simulink model "FB_Controller_UCS"  (R2025b)
settings: Solver=FixedStepDiscrete  StartTime=0.0  StopTime=tspan  FixedStep=dt_sim  RelTol=rel_tol  AbsTol=abs_tol
undefined symbols (not defined in the file): camHardwareDistK, Cimub, const_voltage, dt_control, dt_data, dt_dvl_drr, dt_dvl_vr, dt_sample, dvl, gate1_Pose, initial_joystick_mode_enabled_flag, M_WorldToUCS, manateeOriginPose, pathPoses, redSlalomPoses, rel_CamPose_B, rel_CamPose_B_UCS, rel_CamPose_L, rel_CamPose_L_UCS, rel_CamPose_R, rel_CamPose_R_UCS, save_camera_feed_flag, searchRescueEmojiPose, Sim3dSensor, surveyRepairEmojiPose, use_true_state_flag, whiteSlalomPoses
libraries: sim3dlib x30, visionsinks x3, sim3dcameralib x3, mspsensorlib x1
settings Model: Creator=koryh  LastModifiedBy=Liam

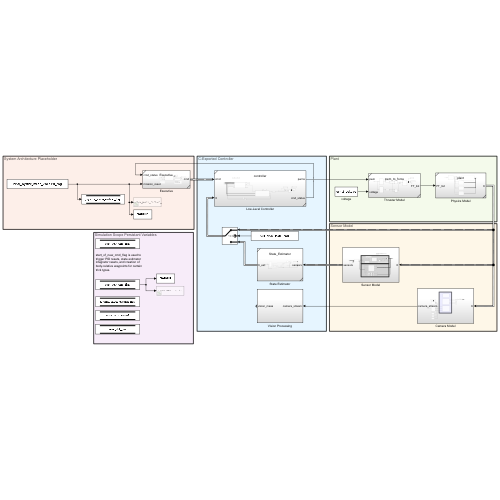
[thumbnail: Simulink's stored preview of the top-level diagram]
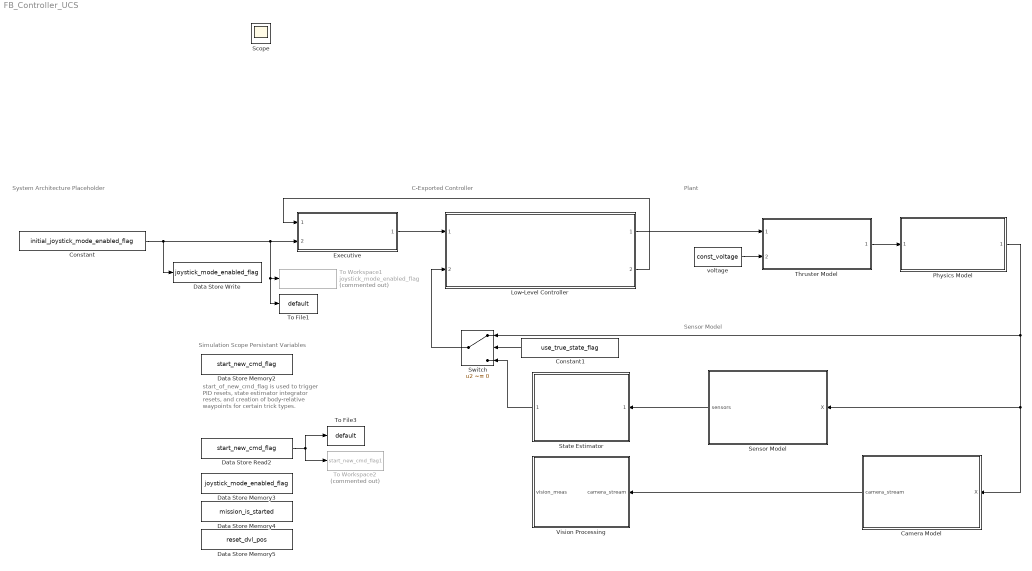
== system FB_Controller_UCS ==
  note: System Architecture Placeholder
  note: Sensor Model
  note: Plant
  note: C-Exported Controller
  note: Simulation Scope Persistant Variables
  note: start_of_new_cmd_flag is used to trigger PID resets, state estimator integrator resets, and creation of body-relative waypoints for certain trick types.
  Camera Model : Subsystem
  Constant : Constant  Value=initial_joystick_mode_enabled_flag
  Constant1 : Constant  Value=use_true_state_flag
  Data Store Memory2 : DataStoreMemory  DataStoreName=start_new_cmd_flag  WriteAfterWriteMsg=warning  InitialValue=true  ShowAdditionalParam=off  OutDataTypeStr=boolean
  Data Store Memory3 : DataStoreMemory  DataStoreName=joystick_mode_enabled_flag  WriteAfterWriteMsg=warning  InitialValue=initial_joystick_mode_enabled_flag  ShowAdditionalParam=off  OutDataTypeStr=boolean
  Data Store Memory4 : DataStoreMemory  DataStoreName=mission_is_started  WriteAfterWriteMsg=warning  InitialValue=false  ShowAdditionalParam=off  OutDataTypeStr=boolean
  Data Store Memory5 : DataStoreMemory  DataStoreName=reset_dvl_pos  WriteAfterWriteMsg=warning  InitialValue=false  ShowAdditionalParam=off  OutDataTypeStr=boolean
  Data Store Read2 : DataStoreRead  DataStoreName=start_new_cmd_flag  IndexOptions=Index vector (dialog)  Indices=1  OutputSizes=1
  Data Store Write : DataStoreWrite  DataStoreName=joystick_mode_enabled_flag  IndexOptions=Index vector (dialog)  Indices=1  OutputSizes=1
  Executive : Subsystem  ReferencedSubsystem=Executive
  Low-Level Controller : Subsystem  ReferencedSubsystem=controller
  Physics Model : Subsystem  ReferencedSubsystem=plant
  Sensor Model : Subsystem
  State Estimator : Subsystem  ReferencedSubsystem=State_Estimator
  Switch : Switch  Criteria=u2 ~= 0  SaturateOnIntegerOverflow=off  InputSameDT=off
  Thruster Model : Subsystem  ReferencedSubsystem=pwm_to_force
  To File1 : ToFile  Filename=default  MatrixName=joystick_mode_enabled_flag  SaveFormat=Timeseries  SampleTime=dt_data
  To File3 : ToFile  Filename=default  MatrixName=start_new_cmd_flag  SaveFormat=Timeseries
  To Workspace1 : ToWorkspace  Commented=on  VariableName=joystick_mode_enabled_flag  SaveFormat=Timeseries  SampleTime=dt_data
  To Workspace2 : ToWorkspace  Commented=on  VariableName=start_new_cmd_flag1  SaveFormat=Timeseries  SampleTime=dt_data
  Vision Processing : Subsystem
  voltage : Constant  Value=const_voltage
  Scope : Scope
      settings: ActiveDisplayYMinimum=-0.048832566475369238  ActiveDisplayYMaximum=0.79721663606048965
  wires:
  voltage/1 -> Thruster Model/2
  Low-Level Controller/1 -> Thruster Model/1
  Thruster Model/1 -> Physics Model/1
  Executive/1 -> Low-Level Controller/1
  Low-Level Controller/2 -> Executive/1
  Physics Model/1 -> Sensor Model/1(X), Camera Model/1(X), Switch/1
  Camera Model/1(camera_stream) -> Vision Processing/1(camera_stream)
  Sensor Model/1(sensors) -> State Estimator/1
  Switch/1 -> Low-Level Controller/2
  Constant1/1 -> Switch/2
  State Estimator/1 -> Switch/3
  Constant/1 -> Data Store Write/1, To File1/1, To Workspace1/1, Executive/2
  Data Store Read2/1 -> To File3/1, To Workspace2/1

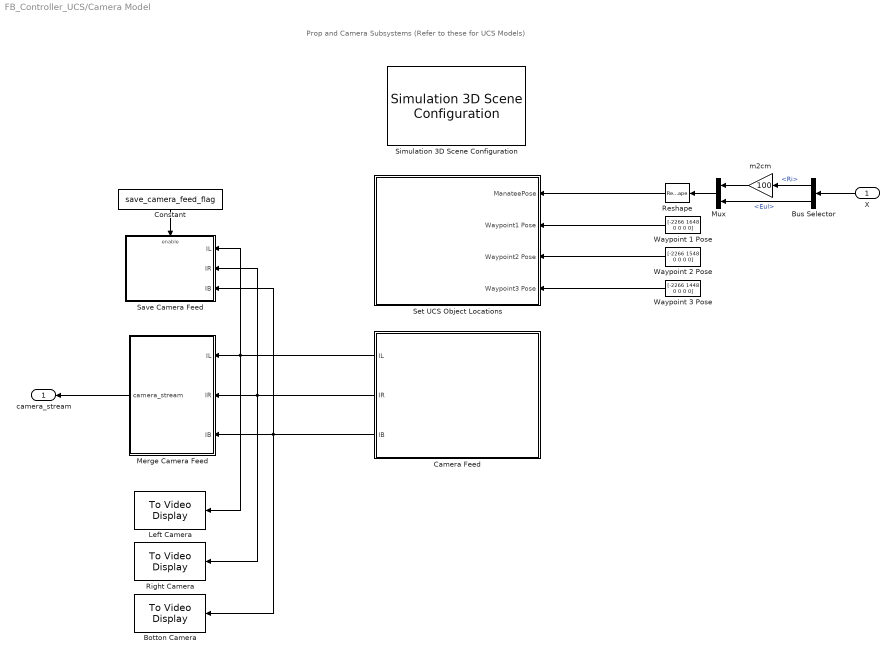
== system FB_Controller_UCS/Camera Model ==
  note: Prop and Camera Subsystems (Refer to these for UCS Models)
  X : Inport
  Botton Camera : visionsinks/To Video Display  windowSizeMode=Normal  openAtMdlStart=off  fullScreen=off  videoWindowX=536805376  videoWindowY=536805376  saveWindowSize=off  videoWindowWidth=1491  videoWindowHeight=834  inputColorFormat=RGB  inputType=Obsolete  imagePorts=One multidimensional signal  OutputDevice=On-screen video monitor  dataOrg=Column-major  isWindowOpen=off
  Bus Selector : BusSelector  OutputSignals=Ri,Eul
  Camera Feed : Subsystem  Priority=1
  Constant : Constant  Value=save_camera_feed_flag
  Left Camera : visionsinks/To Video Display  windowSizeMode=Normal  openAtMdlStart=off  fullScreen=off  videoWindowX=536805376  videoWindowY=536805376  saveWindowSize=off  videoWindowWidth=1491  videoWindowHeight=834  inputColorFormat=RGB  inputType=Obsolete  imagePorts=One multidimensional signal  OutputDevice=On-screen video monitor  dataOrg=Column-major  isWindowOpen=off
  Merge Camera Feed : MATLAB Function  TreatAsAtomicUnit=on
  Mux : Mux  Inputs=2
  Reshape : Reshape  OutputDimensionality=Row vector (2-D)
  Right Camera : visionsinks/To Video Display  windowSizeMode=Normal  openAtMdlStart=off  fullScreen=off  videoWindowX=536805376  videoWindowY=536805376  saveWindowSize=off  videoWindowWidth=1491  videoWindowHeight=834  inputColorFormat=RGB  inputType=Obsolete  imagePorts=One multidimensional signal  OutputDevice=On-screen video monitor  dataOrg=Column-major  isWindowOpen=off
  Save Camera Feed : Subsystem  TreatAsAtomicUnit=on
  Set UCS Object Locations : Subsystem  Priority=1
  Simulation 3D Scene Configuration : sim3dlib/Simulation 3D Scene Configuration  Priority=0  ProjectFormat=Unreal Executable  SceneDesc=Straight road  ProjectName=C:\Users\Liam\OneDrive\Documents\GitHub\SimulinkPlant\DROP UCS PACKAGED BUILD HERE\EllingtonPoolSim.exe  ScenePath=/Game/Olympic_Pool_Course  UEProjPath=C:\Users\Liam\OneDrive\Documents\GitHub\Vision_Sim\Unreal\UnrealProjects\SimulinkCoSimulation\EllingtonPoolSim\EllingtonPoolSim.uproject  EnableOpenDRIVE=off  vehTagList={'Custom';'Scene Origin'}  vehTag=Scene Origin  AttachedCameraRelativeTranslation=[0 0 0]  FreeCameraDefaultInitialTranslation=[-6, 0, 2]  AttachedCameraRelativeRotation=[0 0 0]  FreeCameraDefaultInitialRotation=[0, -15, 0]  ViewpointName=Custom  FreeCameraInitialTranslation=[0, 0, 0]  ViewpointTranslation=[0 0 0]  FreeCameraInitialRotation=[0, 0, 0]  ViewpointRotation=[0 0 0]  OpVisEn=off  Ts=dt_sample  EnableWindow=off  EnableRemoteAccess=off  EnableWeather=off  SunAzimuth=90  SunAltitude=40.0  EnableGeospatialSun=off  Latitude=0  Longitude=0  Date=2023-01-01  Time=10:30:00  GeoTimeZone=-5.0  SunDaylightSaving=off  wind=1  clouds=10  EnableVolumetricClouds=off  CloudCoverage=0  CloudAltitude=6  fog=0  rain=0  RaindropsEffect=off  SnowDensity=0  EnableGeospatial=off  TilesetSource=Earth terrain  UseTrueOrigin=off  OriginHeight=200  OriginLatitude=40.744652  OriginLongitude=-73.988864  MapStyle=Aerial  AdditionalAssetIDs=[]  UseAdvancedSunSky=off  SolarTime=11  TimeZone=-5  Day=21  Month=9  Year=2022  UseDaylightSavingTime=on  DSTStartDay=10  DSTStartMonth=3  DSTEndDay=3  DSTEndMonth=11  DSTSwitchHour=2  sensorTag=MainCamera1  sensorId=1  sensorName=MainCamera1  mountLoc=Origin  offsetFlag=off  tmountOffset=[0, 0, 0]  rmountOffset=[0, 0, 0]  HorizontalResolution=1280  VerticalResolution=720  HorizontalFOV=60  mountPoint=[0 0 0]  mountOrientation=[0 0 0]  aMode=3  ID=1  GeoTrigger=Inactive  ViewNameList={'Custom'}  ViewTranslationList={'[0 0 0]'}  ViewRotationList={'[0 0 0]'}
      settings: LibrarySourceBlock=drivingsim3d/Simulation 3D Scene Configuration
  Waypoint 1 Pose : Constant  Value=[-2266 1648 0 0 0 0]
  Waypoint 2 Pose : Constant  Value=[-2266 1548 0 0 0 0]
  Waypoint 3 Pose : Constant  Value=[-2266 1448 0 0 0 0]
  m2cm : Gain  Gain=100
  camera_stream : Outport
  wires:
  X/1 -> Bus Selector/1
  Bus Selector/1 -> m2cm/1  "<Ri>"
  Bus Selector/2 -> Mux/2  "<Eul>"
  Mux/1 -> Reshape/1
  m2cm/1 -> Mux/1
  Reshape/1 -> Set UCS Object Locations/1(ManateePose)
  Waypoint 1 Pose/1 -> Set UCS Object Locations/2(Waypoint1 Pose)
  Waypoint 2 Pose/1 -> Set UCS Object Locations/3(Waypoint2 Pose)
  Waypoint 3 Pose/1 -> Set UCS Object Locations/4(Waypoint3 Pose)
  Camera Feed/1(IL) -> Save Camera Feed/1(IL), Merge Camera Feed/1(IL), Left Camera/1
  Camera Feed/2(IR) -> Save Camera Feed/2(IR), Merge Camera Feed/2(IR), Right Camera/1
  Camera Feed/3(IB) -> Save Camera Feed/3(IB), Merge Camera Feed/3(IB), Botton Camera/1
  Merge Camera Feed/1(camera_stream) -> camera_stream/1
  Constant/1 -> Save Camera Feed/Enable

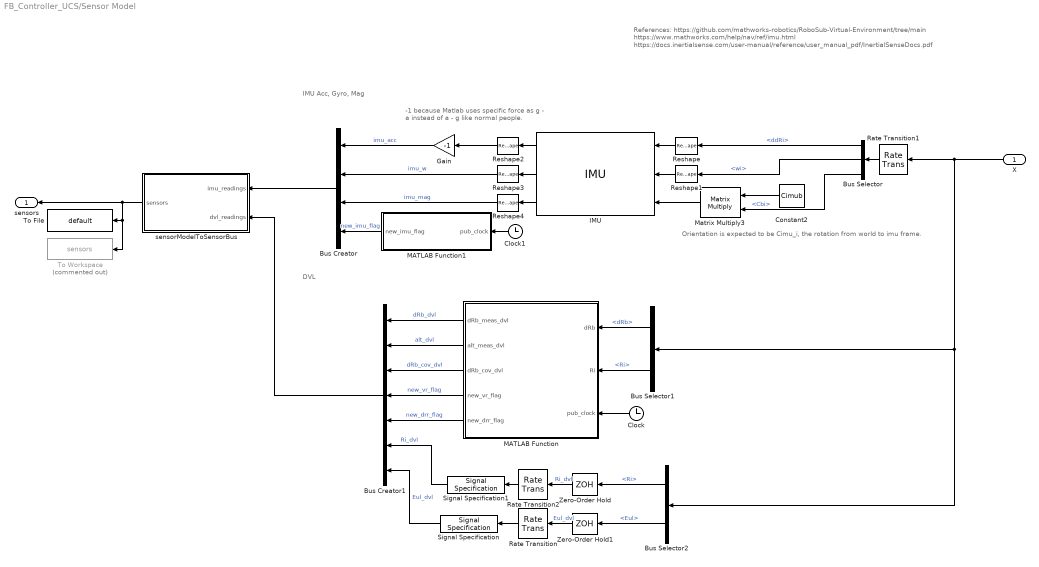
== system FB_Controller_UCS/Sensor Model ==
  note: IMU Acc, Gyro, Mag
  note: -1 because Matlab uses specific force as
      |  g - a instead of a - g like normal people.
  note: Orientation is expected to be Cimu_i, the rotation from world to imu frame.
  note: References:
      | https://github.com/mathworks-robotics/RoboSub-Virtual-Environment/tree/main
      | https://www.mathworks.com/help/nav/ref/imu.html
      | https://docs.inertialsense.com/user-manual/reference/user_manual_pdf/InertialSenseDocs.pdf
  note: DVL
  X : Inport  OutDataTypeStr=Bus: X_bus  SampleTime=dt_control
  Bus Creator : BusCreator  Inputs=4  OutDataTypeStr=Bus: imu_bus
  Bus Creator1 : BusCreator  Inputs=7  OutDataTypeStr=Bus: dvl_bus
  Bus Selector : BusSelector  OutputSignals=ddRi,wi,Cbi
  Bus Selector1 : BusSelector  OutputSignals=dRb,Ri
  Bus Selector2 : BusSelector  OutputSignals=Ri,Eul
  Clock : Clock
  Clock1 : Clock
  Constant2 : Constant  Value=Cimub
  Gain : Gain  Gain=-1
  IMU : mspsensorlib/IMU  DispRefFrame=NED  TemperaturePort=off  Temperature=imu.T  MagneticFieldPort=off  MagneticFieldNED=imu.Bi  MagneticFieldENU=[ -2.4169, 27.5550, 16.0849 ]  SeedDouble=67  SimulateUsing=Interpreted execution  AccelParamsMeasurementRange=imu.acc.meas_range  AccelParamsResolution=imu.acc.res  AccelParamsConstantBias=imu.acc.const_bias  AccelParamsAxesMisalignment=imu.acc.axes_skew  AccelParamsNoiseDensity=imu.acc.vel_rand_walk  AccelParamsBiasInstability=imu.acc.bias_inst  AccelParamsBiasInstabilityNumerator=imu.acc.bias_inst_num_coeffs  AccelParamsBiasInstabilityDenominator=imu.acc.bias_inst_den_coeffs  AccelParamsRandomWalk=imu.acc.acc_rand_walk  AccelParamsNoiseType=double-sided  AccelParamsTemperatureBias=imu.acc.temp_bias  AccelParamsTemperatureScaleFactor=imu.acc.temp_scale_factor  GyroParamsMeasurementRange=imu.gyro.max_read  GyroParamsResolution=imu.gyro.res  GyroParamsConstantBias=imu.gyro.const_bias  GyroParamsAxesMisalignment=imu.gyro.axes_skew  GyroParamsAccelerationBias=imu.gyro.bias_from_acc  GyroParamsNoiseDensity=imu.gyro.angle_rand_walk  GyroParamsBiasInstability=imu.gyro.bias_inst  GyroParamsBiasInstabilityNumerator=imu.gyro.bias_inst_filter_num_coeffs  GyroParamsBiasInstabilityDenominator=imu.gyro.bias_inst_filter_den_coeffs  GyroParamsRandomWalk=imu.gyro.rate_rand_walk  GyroParamsNoiseType=double-sided  GyroParamsTemperatureBias=imu.gyro.temp_bias  GyroParamsTemperatureScaleFactor=imu.gyro.temp_scale_factor  MagParamsMeasurementRange=imu.mag.max_read  MagParamsResolution=imu.mag.res  MagParamsConstantBias=imu.mag.const_bias  MagParamsAxesMisalignment=imu.mag.axes_skew  MagParamsNoiseDensity=imu.mag.white_noise_psd  MagParamsBiasInstability=imu.mag.bias_inst  MagParamsBiasInstabilityNumerator=imu.mag.bias_inst_filter_num_coeffs  MagParamsBiasInstabilityDenominator=imu.mag.bias_isnt_filter_den_coeffs  MagParamsRandomWalk=imu.mag.rand_walk  MagParamsNoiseType=double-sided  MagParamsTemperatureBias=imu.mag.temp_bias  MagParamsTemperatureScaleFactor=imu.mag.temp_scale_factor
  MATLAB Function : MATLAB Function  TreatAsAtomicUnit=on
  MATLAB Function1 : MATLAB Function  TreatAsAtomicUnit=on
  Matrix Multiply3 : Product  Multiplication=Matrix(*)
  Rate Transition : RateTransition  Deterministic=off  OutPortSampleTime=dt_control
  Rate Transition1 : RateTransition  OutPortSampleTime=dt_imu
  Rate Transition2 : RateTransition  Deterministic=off  OutPortSampleTime=dt_control
  Reshape : Reshape  OutputDimensionality=Row vector (2-D)
  Reshape1 : Reshape  OutputDimensionality=Row vector (2-D)
  Reshape2 : Reshape  OutputDimensionality=Column vector (2-D)
  Reshape3 : Reshape  OutputDimensionality=Column vector (2-D)
  Reshape4 : Reshape  OutputDimensionality=Column vector (2-D)
  Signal Specification : SignalSpecification  SampleTime=dt_control
  Signal Specification1 : SignalSpecification  SampleTime=dt_control
  To File : ToFile  Filename=default  MatrixName=sensors  SaveFormat=Timeseries  SampleTime=dt_data
  To Workspace : ToWorkspace  Commented=on  VariableName=sensors  SaveFormat=Timeseries  SampleTime=dt_data
  Zero-Order Hold : ZeroOrderHold  SampleTime=dt_dvl_drr
  Zero-Order Hold1 : ZeroOrderHold  SampleTime=dt_dvl_drr
  sensorModelToSensorBus : MATLAB Function  TreatAsAtomicUnit=on
  sensors : Outport  OutDataTypeStr=Bus: sensor_bus  SampleTime=dt_control
  wires:
  X/1 -> Rate Transition1/1, Bus Selector2/1, Bus Selector1/1
  Reshape/1 -> IMU/1
  Bus Selector/2 -> Reshape1/1  "<wi>"
  IMU/1 -> Reshape2/1
  IMU/2 -> Reshape3/1
  IMU/3 -> Reshape4/1
  Reshape1/1 -> IMU/2
  Bus Selector/1 -> Reshape/1  "<ddRi>"
  Matrix Multiply3/1 -> IMU/3
  Constant2/1 -> Matrix Multiply3/1
  Bus Selector/3 -> Matrix Multiply3/2  "<Cbi>"
  Reshape2/1 -> Gain/1
  Bus Selector1/1 -> MATLAB Function/1(dRb)  "<dRb>"
  Bus Selector1/2 -> MATLAB Function/2(Ri)  "<Ri>"
  sensorModelToSensorBus/1(sensors) -> sensors/1, To Workspace/1, To File/1
  Bus Selector2/2 -> Zero-Order Hold1/1  "<Eul>"
  Rate Transition1/1 -> Bus Selector/1
  Clock/1 -> MATLAB Function/3(pub_clock)
  Clock1/1 -> MATLAB Function1/1(pub_clock)
  Gain/1 -> Bus Creator/1  "imu_acc"
  Reshape3/1 -> Bus Creator/2  "imu_w"
  Reshape4/1 -> Bus Creator/3  "imu_mag"
  MATLAB Function1/1(new_imu_flag) -> Bus Creator/4  "new_imu_flag"
  MATLAB Function/1(dRb_meas_dvl) -> Bus Creator1/1  "dRb_dvl"
  MATLAB Function/2(alt_meas_dvl) -> Bus Creator1/2  "alt_dvl"
  MATLAB Function/3(dRb_cov_dvl) -> Bus Creator1/3  "dRb_cov_dvl"
  MATLAB Function/4(new_vr_flag) -> Bus Creator1/4  "new_vr_flag"
  MATLAB Function/5(new_drr_flag) -> Bus Creator1/5  "new_drr_flag"
  Bus Creator/1 -> sensorModelToSensorBus/1(imu_readings)
  Bus Creator1/1 -> sensorModelToSensorBus/2(dvl_readings)
  Zero-Order Hold/1 -> Rate Transition2/1  "Ri_dvl"
  Signal Specification1/1 -> Bus Creator1/6  "Ri_dvl"
  Signal Specification/1 -> Bus Creator1/7  "Eul_dvl"
  Rate Transition/1 -> Signal Specification/1
  Rate Transition2/1 -> Signal Specification1/1
  Zero-Order Hold1/1 -> Rate Transition/1  "Eul_dvl"
  Bus Selector2/1 -> Zero-Order Hold/1  "<Ri>"

== system FB_Controller_UCS/Vision Processing ==
  camera_stream : Inport
  vision_meas : Outport

== system FB_Controller_UCS/Camera Model/Camera Feed ==
  Simulation 3D Manatee Bottom Camera : sim3dcameralib/Simulation 3D Camera  Priority=1  sensorTag=Sim3dSensor�  sensorId=1  sensorName=Sim3dSensor�  vehTagList={'Scene Origin'}  vehTag=Scene Origin  CoordinateSystem=Default  mountLoc=Origin  offsetFlag=on  tmountOffset=rel_CamPose_B_UCS(1:3) / 100  extTmount=off  rmountOffset=rel_CamPose_B(4:6)  extRmount=off  FocalLength=[2.97 / 0.0028, 2.97 / 0.0028]  OpticalCenter=[960, 540]  ImageSize=[1080, 1920]  RadialDistortion=[camHardwareDistK(1) camHardwareDistK(2) camHardwareDistK(5)]  TangentialDistortion=[camHardwareDistK(3) camHardwareDistK(4)]  SensorSkew=0  VisualizeFieldOfView=on  FieldOfViewRange=61  DepthOutportEnabled=off  SemanticOutportEnabled=off  TransformOutportEnabled=off  SampleTime=dt_sample  mountPoint=[0.23 0 -0.08]  mountOrientation=[0 -1.5707963267949 0]  aMode=5  ID=1
      settings: LibrarySourceBlock=sl3dlib/Simulation 3D/Sensors/Simulation 3D Camera
  Simulation 3D Manatee Left Camera : sim3dcameralib/Simulation 3D Camera  Priority=1  sensorTag=Sim3dSensor�  sensorId=2  sensorName=Sim3dSensor�  vehTagList={'Scene Origin'}  vehTag=Scene Origin  CoordinateSystem=Default  mountLoc=Origin  offsetFlag=on  tmountOffset=rel_CamPose_L_UCS(1:3) / 100  extTmount=off  rmountOffset=rel_CamPose_L(4:6)  extRmount=off  FocalLength=[2.97 / 0.0028, 2.97 / 0.0028]  OpticalCenter=[960, 540]  ImageSize=[1080, 1920]  RadialDistortion=[camHardwareDistK(1) camHardwareDistK(2) camHardwareDistK(5)]  TangentialDistortion=[camHardwareDistK(3) camHardwareDistK(4)]  SensorSkew=0  VisualizeFieldOfView=on  FieldOfViewRange=61  DepthOutportEnabled=off  SemanticOutportEnabled=off  TransformOutportEnabled=off  SampleTime=dt_sample  mountPoint=[0.38 -0.024 0.14]  mountOrientation=[0 0 0]  aMode=5  ID=2
      settings: LibrarySourceBlock=sl3dlib/Simulation 3D/Sensors/Simulation 3D Camera
  Simulation 3D Manatee Right Camera : sim3dcameralib/Simulation 3D Camera  Priority=1  sensorTag=Sim3dSensor�  sensorId=3  sensorName=Sim3dSensor�  vehTagList={'Scene Origin'}  vehTag=Scene Origin  CoordinateSystem=Default  mountLoc=Origin  offsetFlag=on  tmountOffset=rel_CamPose_R_UCS(1:3) / 100  extTmount=off  rmountOffset=rel_CamPose_R(4:6)  extRmount=off  FocalLength=[2.97 / 0.0028, 2.97 / 0.0028]  OpticalCenter=[960, 540]  ImageSize=[1080, 1920]  RadialDistortion=[camHardwareDistK(1) camHardwareDistK(2) camHardwareDistK(5)]  TangentialDistortion=[camHardwareDistK(3) camHardwareDistK(4)]  SensorSkew=0  VisualizeFieldOfView=on  FieldOfViewRange=61  DepthOutportEnabled=off  SemanticOutportEnabled=off  TransformOutportEnabled=off  SampleTime=dt_sample  mountPoint=[0.38 0.024 0.14]  mountOrientation=[0 0 0]  aMode=5  ID=3
      settings: LibrarySourceBlock=sl3dlib/Simulation 3D/Sensors/Simulation 3D Camera
  IL : Outport
  IR : Outport  Port=2
  IB : Outport  Port=3
  wires:
  Simulation 3D Manatee Left Camera/1 -> IL/1
  Simulation 3D Manatee Right Camera/1 -> IR/1
  Simulation 3D Manatee Bottom Camera/1 -> IB/1

== system FB_Controller_UCS/Camera Model/Save Camera Feed ==
  IL : Inport
  IR : Inport  Port=2
  IB : Inport  Port=3
  Enable : EnablePort
  To Workspace Bottom : ToWorkspace  Commented=on  VariableName=cameraBottom_Feed  SampleTime=dt_sample
  To Workspace Left : ToWorkspace  Commented=on  VariableName=cameraLeft_Feed  SampleTime=dt_sample
  To Workspace Right : ToWorkspace  Commented=on  VariableName=cameraRight_Feed  SampleTime=dt_sample
  wires:
  IL/1 -> To Workspace Left/1
  IR/1 -> To Workspace Right/1
  IB/1 -> To Workspace Bottom/1

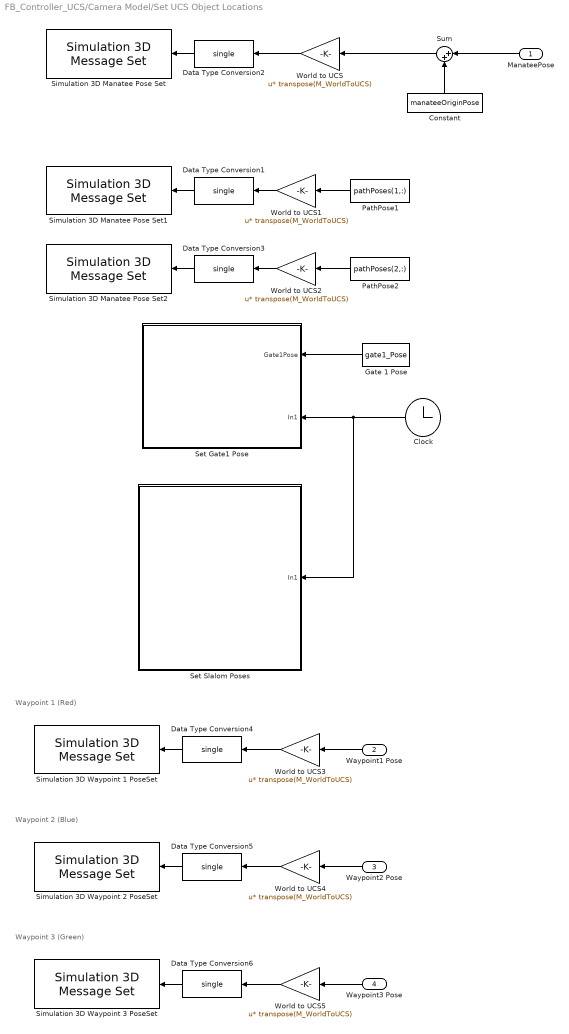
== system FB_Controller_UCS/Camera Model/Set UCS Object Locations ==
  note: Waypoint 1 (Red)
  note: Waypoint 2 (Blue)
  note: Waypoint 3 (Green)
  ManateePose : Inport
  Waypoint1 Pose : Inport  Port=2
  Waypoint2 Pose : Inport  Port=3
  Waypoint3 Pose : Inport  Port=4
  Clock : Clock
      settings: Decimation=dt_sample/dt_sim
  Constant : Constant  Value=manateeOriginPose
  Data Type Conversion{1..6} (6 alike) : DataTypeConversion  OutDataTypeStr=single  SaturateOnIntegerOverflow=off  RndMeth=Floor
  Gate 1 Pose : Constant  Value=gate1_Pose
  PathPose1 : Constant  Value=pathPoses(1,:)
  PathPose2 : Constant  Value=pathPoses(2,:)
  Set Gate1 Pose : Subsystem
  Set Slalom Poses : Subsystem
  Simulation 3D Manatee Pose Set : sim3dlib/Simulation 3D Message Set  Priority=-1  SigName=ManateePoseSet  Ts=dt_sample  aMode=0
      settings: LibrarySourceBlock=aerolibsim3d/Simulation 3D Message Set
  Simulation 3D Manatee Pose Set1 : sim3dlib/Simulation 3D Message Set  Priority=-1  SigName=Path1PoseSet  Ts=dt_sample  aMode=0
      settings: LibrarySourceBlock=aerolibsim3d/Simulation 3D Message Set
  Simulation 3D Manatee Pose Set2 : sim3dlib/Simulation 3D Message Set  Priority=-1  SigName=Path2PoseSet  Ts=dt_sample  aMode=0
      settings: LibrarySourceBlock=aerolibsim3d/Simulation 3D Message Set
  Simulation 3D Waypoint 1 PoseSet : sim3dlib/Simulation 3D Message Set  Priority=-1  SigName=Waypoint1PoseSet  Ts=dt_sample  aMode=0
      settings: LibrarySourceBlock=aerolibsim3d/Simulation 3D Message Set
  Simulation 3D Waypoint 2 PoseSet : sim3dlib/Simulation 3D Message Set  Priority=-1  SigName=Waypoint2PoseSet  Ts=dt_sample  aMode=0
      settings: LibrarySourceBlock=aerolibsim3d/Simulation 3D Message Set
  Simulation 3D Waypoint 3 PoseSet : sim3dlib/Simulation 3D Message Set  Priority=-1  SigName=Waypoint3PoseSet  Ts=dt_sample  aMode=0
      settings: LibrarySourceBlock=aerolibsim3d/Simulation 3D Message Set
  Sum : Sum  Inputs=|++
  World to UCS{,1..5} (6 alike) : Gain  Gain=transpose(M_WorldToUCS)  Multiplication=Matrix(u*K)
  wires:
  Gate 1 Pose/1 -> Set Gate1 Pose/1(Gate1Pose)
  Data Type Conversion2/1 -> Simulation 3D Manatee Pose Set/1
  World to UCS1/1 -> Data Type Conversion1/1
  Data Type Conversion1/1 -> Simulation 3D Manatee Pose Set1/1
  PathPose1/1 -> World to UCS1/1
  World to UCS2/1 -> Data Type Conversion3/1
  Data Type Conversion3/1 -> Simulation 3D Manatee Pose Set2/1
  PathPose2/1 -> World to UCS2/1
  Clock/1 -> Set Slalom Poses/1(In1), Set Gate1 Pose/2(In1)
  World to UCS/1 -> Data Type Conversion2/1
  Waypoint1 Pose/1 -> World to UCS3/1
  Data Type Conversion4/1 -> Simulation 3D Waypoint 1 PoseSet/1
  World to UCS3/1 -> Data Type Conversion4/1
  Waypoint2 Pose/1 -> World to UCS4/1
  Data Type Conversion5/1 -> Simulation 3D Waypoint 2 PoseSet/1
  World to UCS4/1 -> Data Type Conversion5/1
  World to UCS5/1 -> Data Type Conversion6/1
  Waypoint3 Pose/1 -> World to UCS5/1
  Data Type Conversion6/1 -> Simulation 3D Waypoint 3 PoseSet/1
  ManateePose/1 -> Sum/1
  Sum/1 -> World to UCS/1
  Constant/1 -> Sum/2

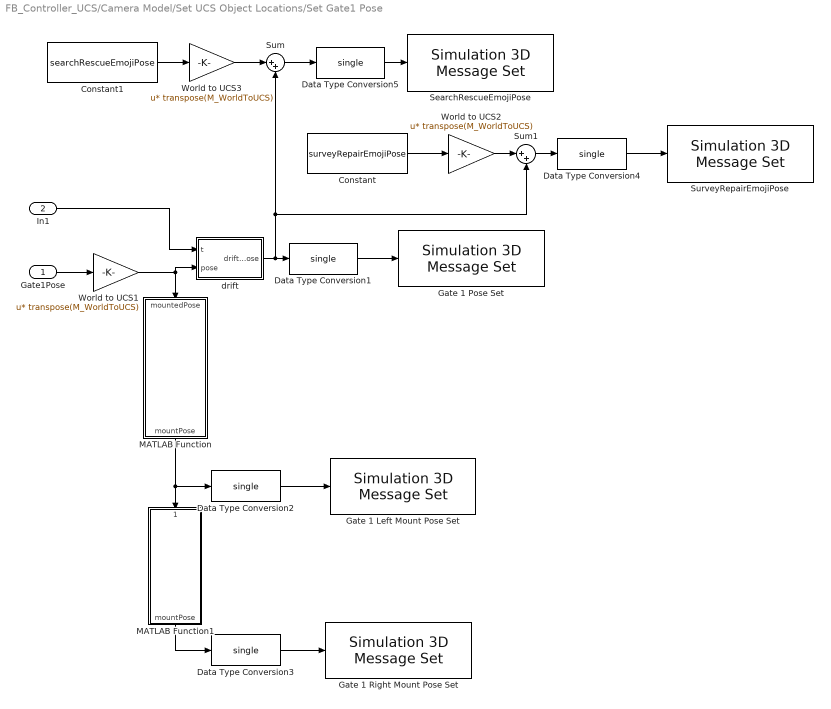
== system FB_Controller_UCS/Camera Model/Set UCS Object Locations/Set Gate1 Pose ==
  Gate1Pose : Inport
  In1 : Inport  Port=2
  Constant : Constant  Value=surveyRepairEmojiPose
  Constant1 : Constant  Value=searchRescueEmojiPose
  Data Type Conversion{1..5} (5 alike) : DataTypeConversion  OutDataTypeStr=single  SaturateOnIntegerOverflow=off  RndMeth=Floor
  Gate 1 Left Mount Pose Set : sim3dlib/Simulation 3D Message Set  Priority=-1  SigName=Gate1LeftMountPoseSet  Ts=dt_sample  aMode=0
      settings: LibrarySourceBlock=aerolibsim3d/Simulation 3D Message Set
  Gate 1 Pose Set : sim3dlib/Simulation 3D Message Set  Priority=-1  SigName=Gate1PoseSet  Ts=dt_sample  aMode=0
      settings: LibrarySourceBlock=aerolibsim3d/Simulation 3D Message Set
  Gate 1 Right Mount Pose Set : sim3dlib/Simulation 3D Message Set  Priority=-1  SigName=Gate1RightMountPoseSet  Ts=dt_sample  aMode=0
      settings: LibrarySourceBlock=aerolibsim3d/Simulation 3D Message Set
  MATLAB Function : MATLAB Function  TreatAsAtomicUnit=on
  MATLAB Function1 : MATLAB Function  TreatAsAtomicUnit=on
  SearchRescueEmojiPose : sim3dlib/Simulation 3D Message Set  Priority=-1  SigName=SearchRescueEmojiPoseSet  Ts=dt_sample  aMode=0
      settings: LibrarySourceBlock=aerolibsim3d/Simulation 3D Message Set
  Sum : Sum  Inputs=|++
  Sum1 : Sum  Inputs=|++
  SurveyRepairEmojiPose : sim3dlib/Simulation 3D Message Set  Priority=-1  SigName=SurveyRepairEmojiPoseSet  Ts=dt_sample  aMode=0
      settings: LibrarySourceBlock=aerolibsim3d/Simulation 3D Message Set
  World to UCS1 : Gain  Gain=transpose(M_WorldToUCS)  Multiplication=Matrix(u*K)
  World to UCS2 : Gain  Gain=transpose(M_WorldToUCS)  Multiplication=Matrix(u*K)
  World to UCS3 : Gain  Gain=transpose(M_WorldToUCS)  Multiplication=Matrix(u*K)
  drift : MATLAB Function  TreatAsAtomicUnit=on
  wires:
  Gate1Pose/1 -> World to UCS1/1
  MATLAB Function/1(mountPose) -> Data Type Conversion2/1, MATLAB Function1/1(leftMountPose)
  Data Type Conversion2/1 -> Gate 1 Left Mount Pose Set/1
  Data Type Conversion3/1 -> Gate 1 Right Mount Pose Set/1
  Data Type Conversion1/1 -> Gate 1 Pose Set/1
  World to UCS1/1 -> drift/2(pose), MATLAB Function/1(mountedPose)
  MATLAB Function1/1(mountPose) -> Data Type Conversion3/1
  Data Type Conversion4/1 -> SurveyRepairEmojiPose/1
  Constant/1 -> World to UCS2/1
  Data Type Conversion5/1 -> SearchRescueEmojiPose/1
  Constant1/1 -> World to UCS3/1
  Sum/1 -> Data Type Conversion5/1
  World to UCS3/1 -> Sum/1
  World to UCS2/1 -> Sum1/1
  Sum1/1 -> Data Type Conversion4/1
  In1/1 -> drift/1(t)
  drift/1(driftPose) -> Data Type Conversion1/1, Sum1/2, Sum/2

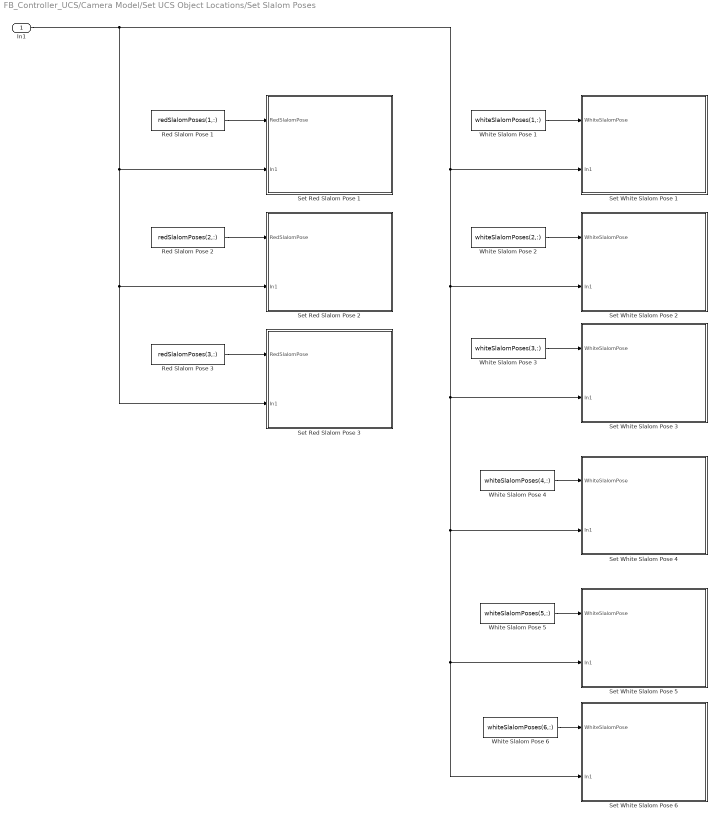
== system FB_Controller_UCS/Camera Model/Set UCS Object Locations/Set Slalom Poses ==
  In1 : Inport
  Red Slalom Pose 1 : Constant  Value=redSlalomPoses(1,:)
  Red Slalom Pose 2 : Constant  Value=redSlalomPoses(2,:)
  Red Slalom Pose 3 : Constant  Value=redSlalomPoses(3,:)
  Set Red Slalom Pose 1 : Subsystem
  Set Red Slalom Pose 2 : Subsystem
  Set Red Slalom Pose 3 : Subsystem
  Set White Slalom Pose 1 : Subsystem
  Set White Slalom Pose 2 : Subsystem
  Set White Slalom Pose 3 : Subsystem
  Set White Slalom Pose 4 : Subsystem
  Set White Slalom Pose 5 : Subsystem
  Set White Slalom Pose 6 : Subsystem
  White Slalom Pose 1 : Constant  Value=whiteSlalomPoses(1,:)
  White Slalom Pose 2 : Constant  Value=whiteSlalomPoses(2,:)
  White Slalom Pose 3 : Constant  Value=whiteSlalomPoses(3,:)
  White Slalom Pose 4 : Constant  Value=whiteSlalomPoses(4,:)
  White Slalom Pose 5 : Constant  Value=whiteSlalomPoses(5,:)
  White Slalom Pose 6 : Constant  Value=whiteSlalomPoses(6,:)
  wires:
  Red Slalom Pose 1/1 -> Set Red Slalom Pose 1/1(RedSlalomPose)
  Red Slalom Pose 2/1 -> Set Red Slalom Pose 2/1(RedSlalomPose)
  Red Slalom Pose 3/1 -> Set Red Slalom Pose 3/1(RedSlalomPose)
  White Slalom Pose 1/1 -> Set White Slalom Pose 1/1(WhiteSlalomPose)
  White Slalom Pose 2/1 -> Set White Slalom Pose 2/1(WhiteSlalomPose)
  White Slalom Pose 3/1 -> Set White Slalom Pose 3/1(WhiteSlalomPose)
  White Slalom Pose 4/1 -> Set White Slalom Pose 4/1(WhiteSlalomPose)
  White Slalom Pose 5/1 -> Set White Slalom Pose 5/1(WhiteSlalomPose)
  White Slalom Pose 6/1 -> Set White Slalom Pose 6/1(WhiteSlalomPose)
  In1/1 -> Set Red Slalom Pose 3/2(In1), Set Red Slalom Pose 2/2(In1), Set Red Slalom Pose 1/2(In1), Set White Slalom Pose 6/2(In1), Set White Slalom Pose 5/2(In1), Set White Slalom Pose 4/2(In1), Set White Slalom Pose 3/2(In1), Set White Slalom Pose 2/2(In1), Set White Slalom Pose 1/2(In1)

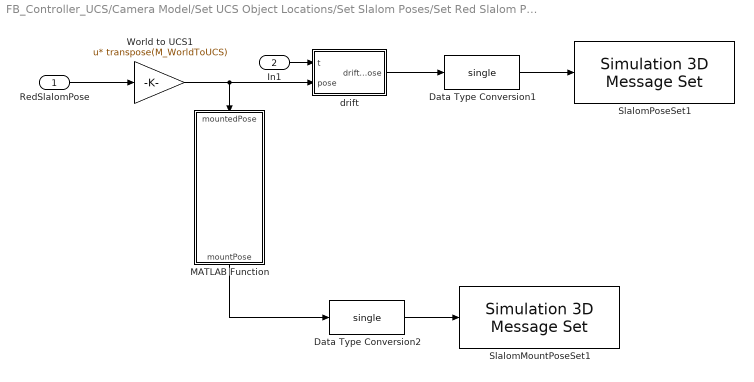
== system FB_Controller_UCS/Camera Model/Set UCS Object Locations/Set Slalom Poses/Set Red Slalom Pose 1 ==
  RedSlalomPose : Inport
  In1 : Inport  Port=2
  Data Type Conversion1 : DataTypeConversion  OutDataTypeStr=single  SaturateOnIntegerOverflow=off  RndMeth=Floor
  Data Type Conversion2 : DataTypeConversion  OutDataTypeStr=single  SaturateOnIntegerOverflow=off  RndMeth=Floor
  MATLAB Function : MATLAB Function  TreatAsAtomicUnit=on
  SlalomMountPoseSet1 : sim3dlib/Simulation 3D Message Set  Priority=-1  SigName=RedSlalom1MountPoseSet  Ts=dt_sample  aMode=0
      settings: LibrarySourceBlock=aerolibsim3d/Simulation 3D Message Set
  SlalomPoseSet1 : sim3dlib/Simulation 3D Message Set  Priority=-1  SigName=RedSlalom1PoseSet  Ts=dt_sample  aMode=0
      settings: LibrarySourceBlock=aerolibsim3d/Simulation 3D Message Set
  World to UCS1 : Gain  Gain=transpose(M_WorldToUCS)  Multiplication=Matrix(u*K)
  drift : MATLAB Function  TreatAsAtomicUnit=on
  wires:
  RedSlalomPose/1 -> World to UCS1/1
  MATLAB Function/1(mountPose) -> Data Type Conversion2/1
  Data Type Conversion2/1 -> SlalomMountPoseSet1/1
  Data Type Conversion1/1 -> SlalomPoseSet1/1
  World to UCS1/1 -> drift/2(pose), MATLAB Function/1(mountedPose)
  drift/1(driftPose) -> Data Type Conversion1/1
  In1/1 -> drift/1(t)

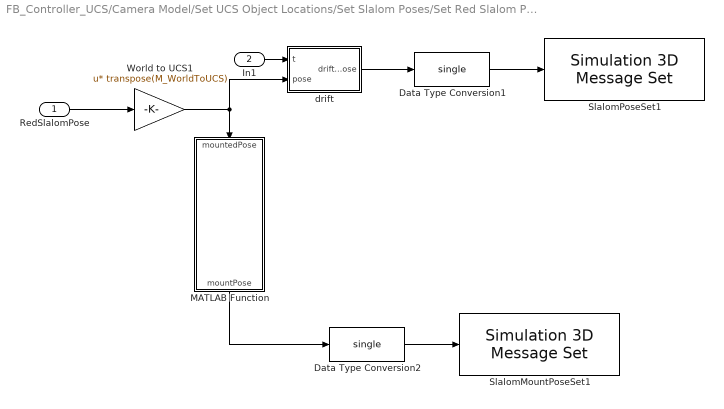
== system FB_Controller_UCS/Camera Model/Set UCS Object Locations/Set Slalom Poses/Set Red Slalom Pose 2 ==
  RedSlalomPose : Inport
  In1 : Inport  Port=2
  Data Type Conversion1 : DataTypeConversion  OutDataTypeStr=single  SaturateOnIntegerOverflow=off  RndMeth=Floor
  Data Type Conversion2 : DataTypeConversion  OutDataTypeStr=single  SaturateOnIntegerOverflow=off  RndMeth=Floor
  MATLAB Function : MATLAB Function  TreatAsAtomicUnit=on
  SlalomMountPoseSet1 : sim3dlib/Simulation 3D Message Set  Priority=-1  SigName=RedSlalom2MountPoseSet  Ts=dt_sample  aMode=0
      settings: LibrarySourceBlock=aerolibsim3d/Simulation 3D Message Set
  SlalomPoseSet1 : sim3dlib/Simulation 3D Message Set  Priority=-1  SigName=RedSlalom2PoseSet  Ts=dt_sample  aMode=0
      settings: LibrarySourceBlock=aerolibsim3d/Simulation 3D Message Set
  World to UCS1 : Gain  Gain=transpose(M_WorldToUCS)  Multiplication=Matrix(u*K)
  drift : MATLAB Function  TreatAsAtomicUnit=on
  wires:
  RedSlalomPose/1 -> World to UCS1/1
  MATLAB Function/1(mountPose) -> Data Type Conversion2/1
  Data Type Conversion2/1 -> SlalomMountPoseSet1/1
  Data Type Conversion1/1 -> SlalomPoseSet1/1
  World to UCS1/1 -> MATLAB Function/1(mountedPose), drift/2(pose)
  In1/1 -> drift/1(t)
  drift/1(driftPose) -> Data Type Conversion1/1

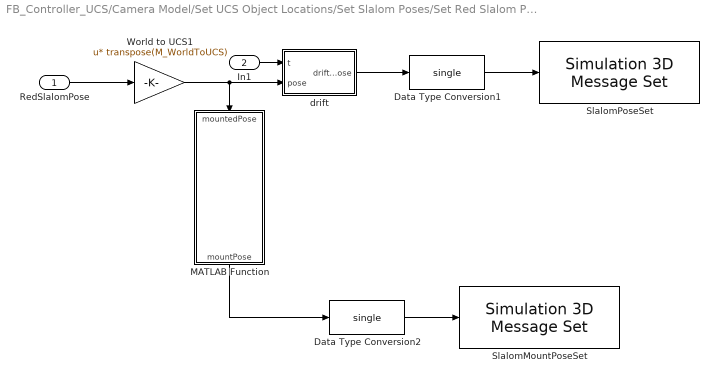
== system FB_Controller_UCS/Camera Model/Set UCS Object Locations/Set Slalom Poses/Set Red Slalom Pose 3 ==
  RedSlalomPose : Inport
  In1 : Inport  Port=2
  Data Type Conversion1 : DataTypeConversion  OutDataTypeStr=single  SaturateOnIntegerOverflow=off  RndMeth=Floor
  Data Type Conversion2 : DataTypeConversion  OutDataTypeStr=single  SaturateOnIntegerOverflow=off  RndMeth=Floor
  MATLAB Function : MATLAB Function  TreatAsAtomicUnit=on
  SlalomMountPoseSet : sim3dlib/Simulation 3D Message Set  Priority=-1  SigName=RedSlalom3MountPoseSet  Ts=dt_sample  aMode=0
      settings: LibrarySourceBlock=aerolibsim3d/Simulation 3D Message Set
  SlalomPoseSet : sim3dlib/Simulation 3D Message Set  Priority=-1  SigName=RedSlalom3PoseSet  Ts=dt_sample  aMode=0
      settings: LibrarySourceBlock=aerolibsim3d/Simulation 3D Message Set
  World to UCS1 : Gain  Gain=transpose(M_WorldToUCS)  Multiplication=Matrix(u*K)
  drift : MATLAB Function  TreatAsAtomicUnit=on
  wires:
  RedSlalomPose/1 -> World to UCS1/1
  MATLAB Function/1(mountPose) -> Data Type Conversion2/1
  Data Type Conversion2/1 -> SlalomMountPoseSet/1
  Data Type Conversion1/1 -> SlalomPoseSet/1
  World to UCS1/1 -> drift/2(pose), MATLAB Function/1(mountedPose)
  In1/1 -> drift/1(t)
  drift/1(driftPose) -> Data Type Conversion1/1

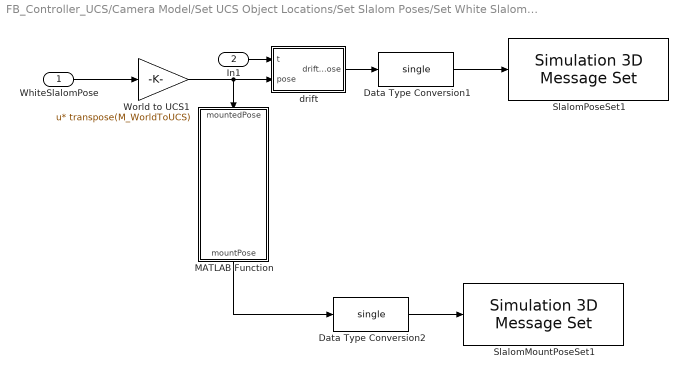
== system FB_Controller_UCS/Camera Model/Set UCS Object Locations/Set Slalom Poses/Set White Slalom Pose 1 ==
  WhiteSlalomPose : Inport
  In1 : Inport  Port=2
  Data Type Conversion1 : DataTypeConversion  OutDataTypeStr=single  SaturateOnIntegerOverflow=off  RndMeth=Floor
  Data Type Conversion2 : DataTypeConversion  OutDataTypeStr=single  SaturateOnIntegerOverflow=off  RndMeth=Floor
  MATLAB Function : MATLAB Function  TreatAsAtomicUnit=on
  SlalomMountPoseSet1 : sim3dlib/Simulation 3D Message Set  Priority=-1  SigName=WhiteSlalom1MountPoseSet  Ts=dt_sample  aMode=0
      settings: LibrarySourceBlock=aerolibsim3d/Simulation 3D Message Set
  SlalomPoseSet1 : sim3dlib/Simulation 3D Message Set  Priority=-1  SigName=WhiteSlalom1PoseSet  Ts=dt_sample  aMode=0
      settings: LibrarySourceBlock=aerolibsim3d/Simulation 3D Message Set
  World to UCS1 : Gain  Gain=transpose(M_WorldToUCS)  Multiplication=Matrix(u*K)
  drift : MATLAB Function  TreatAsAtomicUnit=on
  wires:
  WhiteSlalomPose/1 -> World to UCS1/1
  MATLAB Function/1(mountPose) -> Data Type Conversion2/1
  Data Type Conversion2/1 -> SlalomMountPoseSet1/1
  Data Type Conversion1/1 -> SlalomPoseSet1/1
  World to UCS1/1 -> drift/2(pose), MATLAB Function/1(mountedPose)
  In1/1 -> drift/1(t)
  drift/1(driftPose) -> Data Type Conversion1/1

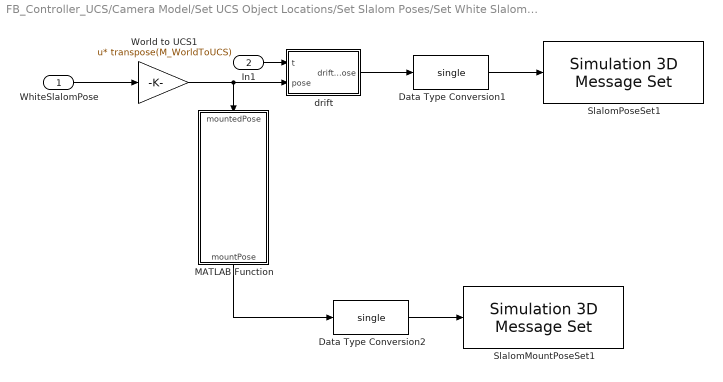
== system FB_Controller_UCS/Camera Model/Set UCS Object Locations/Set Slalom Poses/Set White Slalom Pose 2 ==
  WhiteSlalomPose : Inport
  In1 : Inport  Port=2
  Data Type Conversion1 : DataTypeConversion  OutDataTypeStr=single  SaturateOnIntegerOverflow=off  RndMeth=Floor
  Data Type Conversion2 : DataTypeConversion  OutDataTypeStr=single  SaturateOnIntegerOverflow=off  RndMeth=Floor
  MATLAB Function : MATLAB Function  TreatAsAtomicUnit=on
  SlalomMountPoseSet1 : sim3dlib/Simulation 3D Message Set  Priority=-1  SigName=WhiteSlalom2MountPoseSet  Ts=dt_sample  aMode=0
      settings: LibrarySourceBlock=aerolibsim3d/Simulation 3D Message Set
  SlalomPoseSet1 : sim3dlib/Simulation 3D Message Set  Priority=-1  SigName=WhiteSlalom2PoseSet  Ts=dt_sample  aMode=0
      settings: LibrarySourceBlock=aerolibsim3d/Simulation 3D Message Set
  World to UCS1 : Gain  Gain=transpose(M_WorldToUCS)  Multiplication=Matrix(u*K)
  drift : MATLAB Function  TreatAsAtomicUnit=on
  wires:
  WhiteSlalomPose/1 -> World to UCS1/1
  MATLAB Function/1(mountPose) -> Data Type Conversion2/1
  Data Type Conversion2/1 -> SlalomMountPoseSet1/1
  Data Type Conversion1/1 -> SlalomPoseSet1/1
  World to UCS1/1 -> drift/2(pose), MATLAB Function/1(mountedPose)
  In1/1 -> drift/1(t)
  drift/1(driftPose) -> Data Type Conversion1/1

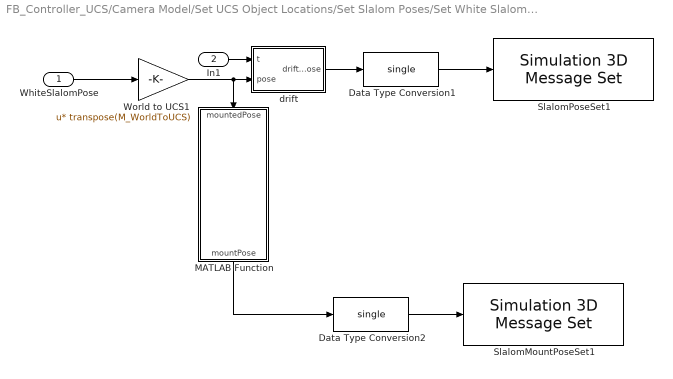
== system FB_Controller_UCS/Camera Model/Set UCS Object Locations/Set Slalom Poses/Set White Slalom Pose 3 ==
  WhiteSlalomPose : Inport
  In1 : Inport  Port=2
  Data Type Conversion1 : DataTypeConversion  OutDataTypeStr=single  SaturateOnIntegerOverflow=off  RndMeth=Floor
  Data Type Conversion2 : DataTypeConversion  OutDataTypeStr=single  SaturateOnIntegerOverflow=off  RndMeth=Floor
  MATLAB Function : MATLAB Function  TreatAsAtomicUnit=on
  SlalomMountPoseSet1 : sim3dlib/Simulation 3D Message Set  Priority=-1  SigName=WhiteSlalom3MountPoseSet  Ts=dt_sample  aMode=0
      settings: LibrarySourceBlock=aerolibsim3d/Simulation 3D Message Set
  SlalomPoseSet1 : sim3dlib/Simulation 3D Message Set  Priority=-1  SigName=WhiteSlalom3PoseSet  Ts=dt_sample  aMode=0
      settings: LibrarySourceBlock=aerolibsim3d/Simulation 3D Message Set
  World to UCS1 : Gain  Gain=transpose(M_WorldToUCS)  Multiplication=Matrix(u*K)
  drift : MATLAB Function  TreatAsAtomicUnit=on
  wires:
  WhiteSlalomPose/1 -> World to UCS1/1
  MATLAB Function/1(mountPose) -> Data Type Conversion2/1
  Data Type Conversion2/1 -> SlalomMountPoseSet1/1
  Data Type Conversion1/1 -> SlalomPoseSet1/1
  World to UCS1/1 -> drift/2(pose), MATLAB Function/1(mountedPose)
  In1/1 -> drift/1(t)
  drift/1(driftPose) -> Data Type Conversion1/1

== system FB_Controller_UCS/Camera Model/Set UCS Object Locations/Set Slalom Poses/Set White Slalom Pose 4 ==
  WhiteSlalomPose : Inport
  In1 : Inport  Port=2
  Data Type Conversion1 : DataTypeConversion  OutDataTypeStr=single  SaturateOnIntegerOverflow=off  RndMeth=Floor
  Data Type Conversion2 : DataTypeConversion  OutDataTypeStr=single  SaturateOnIntegerOverflow=off  RndMeth=Floor
  MATLAB Function : MATLAB Function  TreatAsAtomicUnit=on
  SlalomMountPoseSet1 : sim3dlib/Simulation 3D Message Set  Priority=-1  SigName=WhiteSlalom4MountPoseSet  Ts=dt_sample  aMode=0
      settings: LibrarySourceBlock=aerolibsim3d/Simulation 3D Message Set
  SlalomPoseSet1 : sim3dlib/Simulation 3D Message Set  Priority=-1  SigName=WhiteSlalom4PoseSet  Ts=dt_sample  aMode=0
      settings: LibrarySourceBlock=aerolibsim3d/Simulation 3D Message Set
  World to UCS1 : Gain  Gain=transpose(M_WorldToUCS)  Multiplication=Matrix(u*K)
  drift : MATLAB Function  TreatAsAtomicUnit=on
  wires:
  WhiteSlalomPose/1 -> World to UCS1/1
  MATLAB Function/1(mountPose) -> Data Type Conversion2/1
  Data Type Conversion2/1 -> SlalomMountPoseSet1/1
  Data Type Conversion1/1 -> SlalomPoseSet1/1
  World to UCS1/1 -> drift/2(pose), MATLAB Function/1(mountedPose)
  In1/1 -> drift/1(t)
  drift/1(driftPose) -> Data Type Conversion1/1

== system FB_Controller_UCS/Camera Model/Set UCS Object Locations/Set Slalom Poses/Set White Slalom Pose 5 ==
  WhiteSlalomPose : Inport
  In1 : Inport  Port=2
  Data Type Conversion1 : DataTypeConversion  OutDataTypeStr=single  SaturateOnIntegerOverflow=off  RndMeth=Floor
  Data Type Conversion2 : DataTypeConversion  OutDataTypeStr=single  SaturateOnIntegerOverflow=off  RndMeth=Floor
  MATLAB Function : MATLAB Function  TreatAsAtomicUnit=on
  SlalomMountPoseSet1 : sim3dlib/Simulation 3D Message Set  Priority=-1  SigName=WhiteSlalom5MountPoseSet  Ts=dt_sample  aMode=0
      settings: LibrarySourceBlock=aerolibsim3d/Simulation 3D Message Set
  SlalomPoseSet1 : sim3dlib/Simulation 3D Message Set  Priority=-1  SigName=WhiteSlalom5PoseSet  Ts=dt_sample  aMode=0
      settings: LibrarySourceBlock=aerolibsim3d/Simulation 3D Message Set
  World to UCS1 : Gain  Gain=transpose(M_WorldToUCS)  Multiplication=Matrix(u*K)
  drift : MATLAB Function  TreatAsAtomicUnit=on
  wires:
  WhiteSlalomPose/1 -> World to UCS1/1
  MATLAB Function/1(mountPose) -> Data Type Conversion2/1
  Data Type Conversion2/1 -> SlalomMountPoseSet1/1
  Data Type Conversion1/1 -> SlalomPoseSet1/1
  World to UCS1/1 -> drift/2(pose), MATLAB Function/1(mountedPose)
  In1/1 -> drift/1(t)
  drift/1(driftPose) -> Data Type Conversion1/1

== system FB_Controller_UCS/Camera Model/Set UCS Object Locations/Set Slalom Poses/Set White Slalom Pose 6 ==
  WhiteSlalomPose : Inport
  In1 : Inport  Port=2
  Data Type Conversion1 : DataTypeConversion  OutDataTypeStr=single  SaturateOnIntegerOverflow=off  RndMeth=Floor
  Data Type Conversion2 : DataTypeConversion  OutDataTypeStr=single  SaturateOnIntegerOverflow=off  RndMeth=Floor
  MATLAB Function : MATLAB Function  TreatAsAtomicUnit=on
  SlalomMountPoseSet1 : sim3dlib/Simulation 3D Message Set  Priority=-1  SigName=WhiteSlalom6MountPoseSet  Ts=dt_sample  aMode=0
      settings: LibrarySourceBlock=aerolibsim3d/Simulation 3D Message Set
  SlalomPoseSet1 : sim3dlib/Simulation 3D Message Set  Priority=-1  SigName=WhiteSlalom6PoseSet  Ts=dt_sample  aMode=0
      settings: LibrarySourceBlock=aerolibsim3d/Simulation 3D Message Set
  World to UCS1 : Gain  Gain=transpose(M_WorldToUCS)  Multiplication=Matrix(u*K)
  drift : MATLAB Function  TreatAsAtomicUnit=on
  wires:
  WhiteSlalomPose/1 -> World to UCS1/1
  MATLAB Function/1(mountPose) -> Data Type Conversion2/1
  Data Type Conversion2/1 -> SlalomMountPoseSet1/1
  Data Type Conversion1/1 -> SlalomPoseSet1/1
  World to UCS1/1 -> drift/2(pose), MATLAB Function/1(mountedPose)
  In1/1 -> drift/1(t)
  drift/1(driftPose) -> Data Type Conversion1/1

== matlab function FB_Controller_UCS/Camera Model/Set UCS Object Locations/Set Slalom Poses/Set Red Slalom Pose 3/MATLAB Function ==
  data: mountedPose input; mountPose output; ground_Z parameter
function mountPose = getMountPose(mountedPose,ground_Z)

mountPose = [mountedPose(1) mountedPose(2) (10 - ground_Z) 0 0 mountedPose(6)];

== matlab function FB_Controller_UCS/Camera Model/Set UCS Object Locations/Set Slalom Poses/Set Red Slalom Pose 3/drift ==
  data: t input; pose input; driftPose output
function driftPose = drift(t,pose)
driftPose = toDriftedCoordinates(pose,t);

== matlab function FB_Controller_UCS/Camera Model/Set UCS Object Locations/Set Slalom Poses/Set White Slalom Pose 1/MATLAB Function ==
  data: mountedPose input; mountPose output; ground_Z parameter
function mountPose = getMountPose(mountedPose,ground_Z)

mountPose = [mountedPose(1) mountedPose(2) (10 - ground_Z) 0 0 mountedPose(6)];

== matlab function FB_Controller_UCS/Camera Model/Set UCS Object Locations/Set Slalom Poses/Set White Slalom Pose 1/drift ==
  data: t input; pose input; driftPose output
function driftPose = drift(t,pose)
driftPose = toDriftedCoordinates(pose,t);

== matlab function FB_Controller_UCS/Camera Model/Set UCS Object Locations/Set Slalom Poses/Set White Slalom Pose 2/MATLAB Function ==
  data: mountedPose input; mountPose output; ground_Z parameter
function mountPose = getMountPose(mountedPose,ground_Z)

mountPose = [mountedPose(1) mountedPose(2) (10 - ground_Z) 0 0 mountedPose(6)];

== matlab function FB_Controller_UCS/Camera Model/Set UCS Object Locations/Set Slalom Poses/Set White Slalom Pose 2/drift ==
  data: t input; pose input; driftPose output
function driftPose = drift(t,pose)
driftPose = toDriftedCoordinates(pose,t);

== matlab function FB_Controller_UCS/Camera Model/Set UCS Object Locations/Set Slalom Poses/Set White Slalom Pose 3/MATLAB Function ==
  data: mountedPose input; mountPose output; ground_Z parameter
function mountPose = getMountPose(mountedPose,ground_Z)

mountPose = [mountedPose(1) mountedPose(2) (10 - ground_Z) 0 0 mountedPose(6)];

== matlab function FB_Controller_UCS/Camera Model/Set UCS Object Locations/Set Slalom Poses/Set White Slalom Pose 3/drift ==
  data: t input; pose input; driftPose output
function driftPose = drift(t,pose)
driftPose = toDriftedCoordinates(pose,t);

== matlab function FB_Controller_UCS/Camera Model/Set UCS Object Locations/Set Slalom Poses/Set White Slalom Pose 4/MATLAB Function ==
  data: mountedPose input; mountPose output; ground_Z parameter
function mountPose = getMountPose(mountedPose,ground_Z)

mountPose = [mountedPose(1) mountedPose(2) (10 - ground_Z) 0 0 mountedPose(6)];

== matlab function FB_Controller_UCS/Sensor Model/MATLAB Function1 ==
  settings: updateMethod=DISCRETE  sampleTime=dt_control
  data: pub_clock input; new_imu_flag output; dt_imu parameter
function new_imu_flag = fcn(pub_clock, dt_imu)

persistent last_imu_time

if(isempty(last_imu_time))
    last_imu_time = pub_clock;
end


time_since_last_imu = pub_clock - last_imu_time;

if(time_since_last_imu < dt_imu)
    new_imu_flag = 0;
else
    new_imu_flag = 1;
    last_imu_time = pub_clock;
end

== matlab function FB_Controller_UCS/Camera Model/Set UCS Object Locations/Set Slalom Poses/Set White Slalom Pose 4/drift ==
  data: t input; pose input; driftPose output
function driftPose = drift(t,pose)
driftPose = toDriftedCoordinates(pose,t);

== matlab function FB_Controller_UCS/Camera Model/Set UCS Object Locations/Set Slalom Poses/Set White Slalom Pose 5/MATLAB Function ==
  data: mountedPose input; mountPose output; ground_Z parameter
function mountPose = getMountPose(mountedPose,ground_Z)

mountPose = [mountedPose(1) mountedPose(2) (10 - ground_Z) 0 0 mountedPose(6)];

== matlab function FB_Controller_UCS/Camera Model/Set UCS Object Locations/Set Slalom Poses/Set White Slalom Pose 5/drift ==
  data: t input; pose input; driftPose output
function driftPose = drift(t,pose)
driftPose = toDriftedCoordinates(pose,t);

== matlab function FB_Controller_UCS/Camera Model/Set UCS Object Locations/Set Slalom Poses/Set White Slalom Pose 6/MATLAB Function ==
  data: mountedPose input; mountPose output; ground_Z parameter
function mountPose = getMountPose(mountedPose,ground_Z)

mountPose = [mountedPose(1) mountedPose(2) (10 - ground_Z) 0 0 mountedPose(6)];

== matlab function FB_Controller_UCS/Camera Model/Set UCS Object Locations/Set Slalom Poses/Set White Slalom Pose 6/drift ==
  data: t input; pose input; driftPose output
function driftPose = drift(t,pose)
driftPose = toDriftedCoordinates(pose,t);

== matlab function FB_Controller_UCS/Camera Model/Merge Camera Feed ==
  data: IL input; camera_stream output; IR input; IB input
function camera_stream = mergeCameraFeed(IL,IR,IB)
camera_stream = zeros(3, 1080, 1920, 3);
camera_stream(1,:,:,:) = IL(:,:,:);
camera_stream(2,:,:,:) = IR(:,:,:);
camera_stream(3,:,:,:) = IB(:,:,:);

== matlab function FB_Controller_UCS/Sensor Model/MATLAB Function ==
  settings: updateMethod=DISCRETE  sampleTime=dt_control
  data: dRb input; dRb_meas_dvl output; Ri input; alt_meas_dvl output; dRb_cov_dvl output; dvl parameter; pub_clock input; new_vr_flag output; new_drr_flag output; dt_dvl_vr parameter; dt_dvl_drr parameter
function [dRb_meas_dvl, alt_meas_dvl, dRb_cov_dvl, new_vr_flag, new_drr_flag] = dvl_sim(dRb, Ri,dvl, pub_clock, dt_dvl_vr, dt_dvl_drr)
%{
Model from this repository:
https://github.com/mathworks-robotics/RoboSub-Virtual-Environment/
Need to modify this to give erroneous or no reading when ground lock is
available.

Also need to add noise to the altitude measurement and determine if it
needs modification based on attitude.
%}

persistent last_drr_time
persistent last_vr_time

if(isempty(last_drr_time))
    last_drr_time = pub_clock;
end
if(isempty(last_vr_time))
    last_vr_time = pub_clock;
end

time_since_last_drr = pub_clock - last_drr_time;
time_since_last_vr = pub_clock - last_vr_time;
if(time_since_last_drr < dt_dvl_drr)
    new_drr_flag = 0;
else
    new_drr_flag = 1;
    last_drr_time = pub_clock;
end
if(time_since_last_vr < dt_dvl_vr)
    new_vr_flag = 0;
else
    new_vr_flag = 1;
    last_vr_time = pub_clock;
end



%get altitude (assumes Ri is measured from the robot's starting depth
true_depth = dvl.start_depth + Ri(3); 
true_alt = dvl.pool_depth - true_depth;
alt_meas_dvl = true_alt;

%bias for velocity measurements
persistent bias
if isempty(bias)
    bias = zeros(3,1);
end


% ---------------- Update bias (Gauss-Markov) ----------------
if dvl.bias_tau > 0 && dvl.bias_sigma_ss > 0
    % Discrete-time OU: b_{k+1} = (1 - dt/tau) b_k + sqrt(2*sigma^2*dt/tau) * w
    a = max(0.0, 1.0 - dvl.bias_dt/dvl.bias_tau);
    q = sqrt(max(0.0, 2.0*dvl.bias_sigma_ss^2*dvl.bias_dt/dvl.bias_tau));
    bias = a*bias + q * randn(3,1);
else
    bias = zeros(3,1);
end

% ---------------- Add noise & bias ----------------
noise = dvl.noise_sigma .* randn(3,1);    % white noise
dRb_meas_dvl = dRb + bias + noise;

dRb_cov_dvl = diag([dvl.noise_sigma].^2);

== matlab function FB_Controller_UCS/Sensor Model/sensorModelToSensorBus ==
  settings: updateMethod=DISCRETE  sampleTime=dt_control
  data: imu_readings input; sensors output Bus: sensor_bus; dvl_readings input
function sensors = fcn(imu_readings, dvl_readings)

sensors = sensorModelToSensorBus(imu_readings, dvl_readings);

== matlab function FB_Controller_UCS/Camera Model/Set UCS Object Locations/Set Gate1 Pose/MATLAB Function ==
  data: mountedPose input; mountPose output; ground_Z parameter
function mountPose = getMountPose(mountedPose,ground_Z)

mountPose = [mountedPose(1) mountedPose(2) (10 - ground_Z) 0 0 mountedPose(6)];

== matlab function FB_Controller_UCS/Camera Model/Set UCS Object Locations/Set Gate1 Pose/MATLAB Function1 ==
  data: leftMountPose input; mountPose output
function mountPose = getMountPose(leftMountPose)

phi = leftMountPose(6) * pi / 180 + pi / 2;
xAdjust = 307 * cos(phi);
yAdjust = 307 * sin(phi);

mountPose = [(leftMountPose(1) + xAdjust) (leftMountPose(2) + yAdjust) leftMountPose(3) 0 0 leftMountPose(6)];

== matlab function FB_Controller_UCS/Camera Model/Set UCS Object Locations/Set Gate1 Pose/drift ==
  data: t input; pose input; driftPose output
function driftPose = drift(t,pose)
driftPose = toDriftedCoordinates(pose,t);

== matlab function FB_Controller_UCS/Camera Model/Set UCS Object Locations/Set Slalom Poses/Set Red Slalom Pose 1/MATLAB Function ==
  data: mountedPose input; mountPose output; ground_Z parameter
function mountPose = getMountPose(mountedPose,ground_Z)

mountPose = [mountedPose(1) mountedPose(2) (10 - ground_Z) 0 0 mountedPose(6)];

== matlab function FB_Controller_UCS/Camera Model/Set UCS Object Locations/Set Slalom Poses/Set Red Slalom Pose 1/drift ==
  data: t input; pose input; driftPose output
function driftPose = drift(t,pose)
driftPose = toDriftedCoordinates(pose,t);

== matlab function FB_Controller_UCS/Camera Model/Set UCS Object Locations/Set Slalom Poses/Set Red Slalom Pose 2/MATLAB Function ==
  data: mountedPose input; mountPose output; ground_Z parameter
function mountPose = getMountPose(mountedPose,ground_Z)

mountPose = [mountedPose(1) mountedPose(2) (10 - ground_Z) 0 0 mountedPose(6)];

== matlab function FB_Controller_UCS/Camera Model/Set UCS Object Locations/Set Slalom Poses/Set Red Slalom Pose 2/drift ==
  data: t input; pose input; driftPose output
function driftPose = drift(t,pose)
driftPose = toDriftedCoordinates(pose,t);
